simulink model "Environment"  (R2013a)
settings: Solver=ode45  StartTime=0.0  StopTime=10.0  RelTol=1e-3
model workspace (MATLAB code in the model file):
  | switch(Env)
  |    case 'Pikes Peak'
  |       load Evn_Pikes_Peak;
  |    case 'IOM'
  |       load Evn_IOM;
  |    otherwise
  |       load Environment
  | end
values from neighbouring files (symbols this model uses):
  altx = [0 1 2 3 4 5 6 7 8 9 10 11 ... (6827 elements, 6827x1)]    [Copy_of_Environment.mat]    (also in Environment.mat)
  alty = [2872.8 2872.86 2872.88 2872.81 2872.76 2872.71 2872.66 2872.62 2872.6 2872.58 2872.58 2872.57 ... (6827 elements, 6827x1)]    [Copy_of_Environment.mat]    (also in Environment.mat)
  g = 9.81    [Chassis.mat]    (also in Copy_of_Environment.mat = 9.80665; Environment.mat = 9.80665)
  L = 6500    [Copy_of_Environment.mat]    (also in Environment.mat = 0.0065)
  M = 28.9644    [Copy_of_Environment.mat]    (also in Environment.mat)
  P0 = 100000    [Copy_of_Environment.mat]    (also in Environment.mat)
  R = 8.31432    [Copy_of_Environment.mat]    (also in Environment.mat)
  T0 = 288    [Copy_of_Environment.mat]    (also in Environment.mat = 300)
settings Model: Creator=Nathan  LastModifiedBy=Nathan

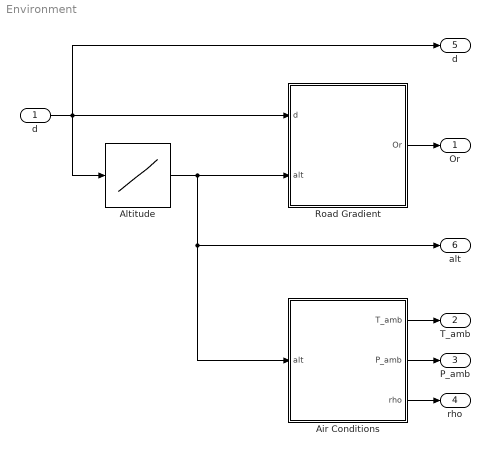
== system Environment ==
  d : Inport
  Air Conditions : Subsystem
  Altitude : Lookup_n-D  NumberOfTableDimensions=1  BreakpointsForDimension1=altx  Table=alty  ExtrapMethod=Clip  DiagnosticForOutOfRangeInput=Warning  UseLastTableValue=on  RndMeth=Simplest  InputSameDT=on
  Road Gradient : Subsystem
  Or : Outport
  T_amb : Outport  Port=2
  P_amb : Outport  Port=3
  rho : Outport  Port=4
  "d " : Outport  Port=5
  alt : Outport  Port=6
  wires:
  d/1 -> "d "/1, Road Gradient/1(d), Altitude/1
  Road Gradient/1(Or) -> Or/1
  Altitude/1 -> alt/1, Air Conditions/1(alt), Road Gradient/2(alt)
  Air Conditions/1("T_amb ") -> T_amb/1
  Air Conditions/2(P_amb) -> P_amb/1
  Air Conditions/3(rho) -> rho/1

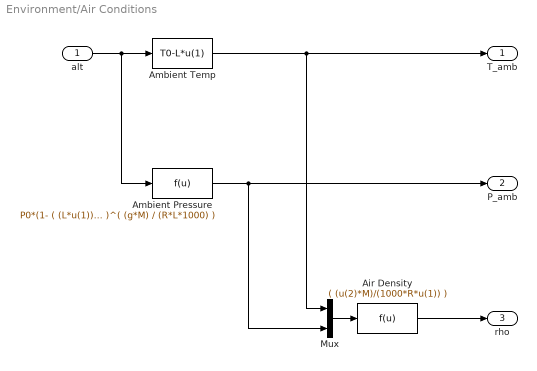
== system Environment/Air Conditions ==
  alt : Inport
  Air Density : Fcn  Expr=( (u(2)*M)/(1000*R*u(1)) )
  Ambient Pressure : Fcn  Expr=P0*(1- ( (L*u(1))/(T0) ) )^( (g*M) / (R*L*1000) )
  Ambient Temp : Fcn  Expr=T0-L*u(1)
  Mux : Mux  Inputs=2
  "T_amb " : Outport
  P_amb : Outport  Port=2
  rho : Outport  Port=3
  wires:
  alt/1 -> Ambient Pressure/1, Ambient Temp/1
  Ambient Temp/1 -> Mux/1, "T_amb "/1
  Ambient Pressure/1 -> Mux/2, P_amb/1
  Mux/1 -> Air Density/1
  Air Density/1 -> rho/1

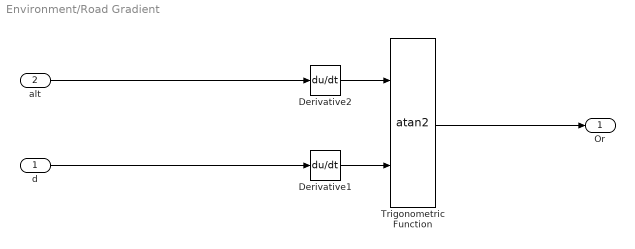
== system Environment/Road Gradient ==
  d : Inport
  alt : Inport  Port=2
  Derivative1 : Derivative
  Derivative2 : Derivative
  Trigonometric Function : Trigonometry  Operator=atan2
  Or : Outport
  wires:
  alt/1 -> Derivative2/1
  Trigonometric Function/1 -> Or/1
  Derivative1/1 -> Trigonometric Function/2
  d/1 -> Derivative1/1
  Derivative2/1 -> Trigonometric Function/1
